simulink model "IEEE_39_bus_steady_state"  (R2021b)
settings: Solver=ode3  StartTime=0.0  StopTime=10  FixedStep=Ts  MaxStep=1/60  RelTol=1e-2  AbsTol=1e-1
PreLoadFcn:
  | Ts=50e-6; ssn_ieee39_params; dec=20;
InitFcn:
  | Ts=50e-6; ssn_ieee39_params; dec=20;
values from neighbouring files (symbols this model uses):
  f = 50    [ssn_ieee39_params_ctrl.m]
  fNom = f    (= 60)    [ssn_ieee39_params_ctrl.m]
  ILR = 5.02    [ssn_ieee39_params_ctrl.m]
  IQMIN = 0.1    [ssn_ieee39_params_ctrl.m]
  ISCLIM = 1    [ssn_ieee39_params_ctrl.m]
  ITFpu = 1.10    (= 1.1)    [ssn_ieee39_params_ctrl.m]
  K = 1    [ssn_ieee39_params_ctrl.m]
  K1 = 1    [ssn_ieee39_params_ctrl.m]
  K2 = 2    [ssn_ieee39_params_ctrl.m]
  KCL = 1.04    [ssn_ieee39_params_ctrl.m]
  KFB = 0    [ssn_ieee39_params_ctrl.m]
  KFF = 1    [ssn_ieee39_params_ctrl.m]
  KFIX = 1    [ssn_ieee39_params_ctrl.m]
  KG = 1    [ssn_ieee39_params_ctrl.m]
  KIA = 59.91    [ssn_ieee39_params_ctrl.m]
  KIOEX = 0.0303    [ssn_ieee39_params_ctrl.m]
  KIUEX = 0.0303    [ssn_ieee39_params_ctrl.m]
  KIUOEX = 1    [ssn_ieee39_params_ctrl.m]
  KIUUEX = 1    [ssn_ieee39_params_ctrl.m]
  KLR = 22.47    [ssn_ieee39_params_ctrl.m]
  KM = 1    [ssn_ieee39_params_ctrl.m]
  KOEL = 0.24    [ssn_ieee39_params_ctrl.m]
  Kp = 1    [ssn_ieee39_params_ctrl.m]
  KPA = 30    [ssn_ieee39_params_ctrl.m]
  KPOEL = 1    [ssn_ieee39_params_ctrl.m]
  KPOEX = 0    [ssn_ieee39_params_ctrl.m]
  KPUEX = 0    [ssn_ieee39_params_ctrl.m]
  KSCALE = 0.319    [ssn_ieee39_params_ctrl.m]
  KUF = 0    [ssn_ieee39_params_ctrl.m]
  KUI = 0.001    [ssn_ieee39_params_ctrl.m]
  KUL = 0.24    [ssn_ieee39_params_ctrl.m]
  s = 10    [ssn_ieee39_params_ctrl.m]
  TA = 0.01    [ssn_ieee39_params_ctrl.m]
  Tadj = 0    [ssn_ieee39_params_ctrl.m]
  taps = [1 1 1.07 1.07 1.009 1.025 1 1.025 1.025 1.025]*1    [ssn_ieee39_params_ctrl.m]
  TF = 0.02    [ssn_ieee39_params_ctrl.m]
  TG = 0.024    [ssn_ieee39_params_ctrl.m]
  TINV = 0    [ssn_ieee39_params_ctrl.m]
  TIT = 0.1    [ssn_ieee39_params_ctrl.m]
  TL_10_11_len = 14    [ssn_ieee39_params_ctrl.m]
  TL_10_13_len = 14    [ssn_ieee39_params_ctrl.m]
  TL_13_14_len = 32    [ssn_ieee39_params_ctrl.m]
  TL_14_15_len = 70    [ssn_ieee39_params_ctrl.m]
  TL_15_16_len = 31.5    [ssn_ieee39_params_ctrl.m]
  TL_16_17_len = 26    [ssn_ieee39_params_ctrl.m]
  TL_16_19_len = 61    [ssn_ieee39_params_ctrl.m]
  TL_16_21_len = 46    [ssn_ieee39_params_ctrl.m]
  TL_16_24_len = 15    [ssn_ieee39_params_ctrl.m]
  TL_17_18_len = 26    [ssn_ieee39_params_ctrl.m]
  TL_17_27_len = 59    [ssn_ieee39_params_ctrl.m]
  TL_1_2_len = 134    [ssn_ieee39_params_ctrl.m]
  TL_1_39_len = 105    [ssn_ieee39_params_ctrl.m]
  TL_21_22_len = 47    [ssn_ieee39_params_ctrl.m]
  TL_22_23_len = 33    [ssn_ieee39_params_ctrl.m]
  TL_24_23_len = 88    [ssn_ieee39_params_ctrl.m]
  TL_25_26_len = 101    [ssn_ieee39_params_ctrl.m]
  TL_26_27_len = 46.5    [ssn_ieee39_params_ctrl.m]
  TL_26_28_len = 151    [ssn_ieee39_params_ctrl.m]
  TL_26_29_len = 200    [ssn_ieee39_params_ctrl.m]
  TL_28_29_len = 48    [ssn_ieee39_params_ctrl.m]
  TL_2_25_len = 28    [ssn_ieee39_params_ctrl.m]
  TL_2_2_len = 49    [ssn_ieee39_params_ctrl.m]
  TL_3_18_len = 42    [ssn_ieee39_params_ctrl.m]
  TL_3_4_len = 53    [ssn_ieee39_params_ctrl.m]
  TL_4_14_len = 33    [ssn_ieee39_params_ctrl.m]
  TL_4_5_len = 32.5    [ssn_ieee39_params_ctrl.m]
  TL_5_6_len = 14    [ssn_ieee39_params_ctrl.m]
  TL_5_8_len = 32    [ssn_ieee39_params_ctrl.m]
  TL_6_11_len = 26.5    [ssn_ieee39_params_ctrl.m]
  TL_6_7_len = 25.5    [ssn_ieee39_params_ctrl.m]
  TL_7_8_len = 15    [ssn_ieee39_params_ctrl.m]
  TL_8_9_len = 93    [ssn_ieee39_params_ctrl.m]
  TL_9_39_len = 136    [ssn_ieee39_params_ctrl.m]
  TOEL = 5.00    (= 5)    [ssn_ieee39_params_ctrl.m]
  TQREF = 0    [ssn_ieee39_params_ctrl.m]
  TQSCL = 0.012    [ssn_ieee39_params_ctrl.m]
  Ts_PMU = 1/1000    (= 0.001)    [ssn_ieee39_params_ctrl.m]
  TU1 = 0    [ssn_ieee39_params_ctrl.m]
  TU2 = 0    [ssn_ieee39_params_ctrl.m]
  TU3 = 0    [ssn_ieee39_params_ctrl.m]
  TU4 = 0    [ssn_ieee39_params_ctrl.m]
  TUL = 0    [ssn_ieee39_params_ctrl.m]
  TUP = 0.050    (= 0.05)    [ssn_ieee39_params_ctrl.m]
  TUQ = .005    (= 0.005)    [ssn_ieee39_params_ctrl.m]
  TUV = 0.2    [ssn_ieee39_params_ctrl.m]
  VAAMAX = VAMAX    (= 7.05)    [ssn_ieee39_params_ctrl.m]
  VAMAX = 7.05    [ssn_ieee39_params_ctrl.m]
  VAMIN = -6.11    [ssn_ieee39_params_ctrl.m]
  VBMAX = 999    [ssn_ieee39_params_ctrl.m]
  VF = 0    [ssn_ieee39_params_ctrl.m]
  VFB = 0    [ssn_ieee39_params_ctrl.m]
  VMMAX = 7.05    [ssn_ieee39_params_ctrl.m]
  VMMIN = -6.11    [ssn_ieee39_params_ctrl.m]
  VOELmax1 = 0.2353    [ssn_ieee39_params_ctrl.m]
  VOELmax2 = 0.0    (= 0)    [ssn_ieee39_params_ctrl.m]
  VOELmin1 = -0.24    [ssn_ieee39_params_ctrl.m]
  VOELmin2 = -1.0    (= -1)    [ssn_ieee39_params_ctrl.m]
  VRMAX = 7.05    [ssn_ieee39_params_ctrl.m]
  VRMIN = -6.11    [ssn_ieee39_params_ctrl.m]
  VSCLmax = 0.20    (= 0.2)    [ssn_ieee39_params_ctrl.m]
  VSCLmin = -0.10    (= -0.1)    [ssn_ieee39_params_ctrl.m]
  VUELmax1 = 1    [ssn_ieee39_params_ctrl.m]
  VUELmax2 = 1    [ssn_ieee39_params_ctrl.m]
  VUELmin1 = -1    [ssn_ieee39_params_ctrl.m]
  VUELmin2 = -1    [ssn_ieee39_params_ctrl.m]
  VUImax = 1    [ssn_ieee39_params_ctrl.m]
  VUImin = -1    [ssn_ieee39_params_ctrl.m]
undefined symbols (not defined in the file or in its folder): D1, Delta, MOV_segment9, powergui
libraries: spsThreePhaseVIMeasurementLib x43, slpidlib x40, op_dpl_lib x32, powerlib_extras x30, simulink_extras x20, spsST2AModel x20, spsThreePhaseParallelRLCLoadLib x20, spsThreePhaseTransformerTwoWindingsLib x13, spsSynchronousMachinepuStandardLib x10, simulink x10, spsPower3phInstantaneousLib x10, spsThreePhasePISectionLineLib x4
(part 3 of 15)

== system IEEE_39_bus_steady_state/powergui ==
  note: Graphical user interface for the analysis of
      | Simscape Power Systems (Specialized Technology) circuits.
      | Place the Powergui block in the top-level of your model and double-click
      | on it to open the GUI.
  EquivalentModel1 : Subsystem
      mask init:
      | S  = GetDataForEquivalentModel('Discrete',gcbh);
      mask Display:
      | color('red')
      | disp('EQUIVALENT CIRCUIT\nDiscrete')
  EquivalentModel10 : Subsystem
      mask init:
      | S  = GetDataForEquivalentModel('Discrete',gcbh);
      mask Display:
      | color('red')
      | disp('EQUIVALENT CIRCUIT\nDiscrete')
  EquivalentModel11 : Subsystem
      mask init:
      | S  = GetDataForEquivalentModel('Discrete',gcbh);
      mask Display:
      | color('red')
      | disp('EQUIVALENT CIRCUIT\nDiscrete')
  EquivalentModel12 : Subsystem
      mask init:
      | S  = GetDataForEquivalentModel('Discrete',gcbh);
      mask Display:
      | color('red')
      | disp('EQUIVALENT CIRCUIT\nDiscrete')
  EquivalentModel13 : Subsystem
      mask init:
      | S  = GetDataForEquivalentModel('Discrete',gcbh);
      mask Display:
      | color('red')
      | disp('EQUIVALENT CIRCUIT\nDiscrete')
  EquivalentModel14 : Subsystem
      mask init:
      | S  = GetDataForEquivalentModel('Discrete',gcbh);
      mask Display:
      | color('red')
      | disp('EQUIVALENT CIRCUIT\nDiscrete')
  EquivalentModel15 : Subsystem
      mask init:
      | S  = GetDataForEquivalentModel('Discrete',gcbh);
      mask Display:
      | color('red')
      | disp('EQUIVALENT CIRCUIT\nDiscrete')
  EquivalentModel16 : Subsystem
      mask init:
      | S  = GetDataForEquivalentModel('Discrete',gcbh);
      mask Display:
      | color('red')
      | disp('EQUIVALENT CIRCUIT\nDiscrete')
  EquivalentModel17 : Subsystem
      mask init:
      | S  = GetDataForEquivalentModel('Discrete',gcbh);
      mask Display:
      | color('red')
      | disp('EQUIVALENT CIRCUIT\nDiscrete')
  EquivalentModel18 : Subsystem
      mask init:
      | S  = GetDataForEquivalentModel('Discrete',gcbh);
      mask Display:
      | color('red')
      | disp('EQUIVALENT CIRCUIT\nDiscrete')
  EquivalentModel19 : Subsystem
      mask init:
      | S  = GetDataForEquivalentModel('Discrete',gcbh);
      mask Display:
      | color('red')
      | disp('EQUIVALENT CIRCUIT\nDiscrete')
  EquivalentModel2 : Subsystem
      mask init:
      | S  = GetDataForEquivalentModel('Discrete',gcbh);
      mask Display:
      | color('red')
      | disp('EQUIVALENT CIRCUIT\nDiscrete')
  EquivalentModel20 : Subsystem
      mask init:
      | S  = GetDataForEquivalentModel('Discrete',gcbh);
      mask Display:
      | color('red')
      | disp('EQUIVALENT CIRCUIT\nDiscrete')
  EquivalentModel21 : Subsystem
      mask init:
      | S  = GetDataForEquivalentModel('Discrete',gcbh);
      mask Display:
      | color('red')
      | disp('EQUIVALENT CIRCUIT\nDiscrete')
  EquivalentModel22 : Subsystem
      mask init:
      | S  = GetDataForEquivalentModel('Discrete',gcbh);
      mask Display:
      | color('red')
      | disp('EQUIVALENT CIRCUIT\nDiscrete')
  EquivalentModel23 : Subsystem
      mask init:
      | S  = GetDataForEquivalentModel('Discrete',gcbh);
      mask Display:
      | color('red')
      | disp('EQUIVALENT CIRCUIT\nDiscrete')
  EquivalentModel24 : Subsystem
      mask init:
      | S  = GetDataForEquivalentModel('Discrete',gcbh);
      mask Display:
      | color('red')
      | disp('EQUIVALENT CIRCUIT\nDiscrete')
  EquivalentModel25 : Subsystem
      mask init:
      | S  = GetDataForEquivalentModel('Discrete',gcbh);
      mask Display:
      | color('red')
      | disp('EQUIVALENT CIRCUIT\nDiscrete')
  EquivalentModel26 : Subsystem
      mask init:
      | S  = GetDataForEquivalentModel('Discrete',gcbh);
      mask Display:
      | color('red')
      | disp('EQUIVALENT CIRCUIT\nDiscrete')
  EquivalentModel3 : Subsystem
      mask init:
      | S  = GetDataForEquivalentModel('Discrete',gcbh);
      mask Display:
      | color('red')
      | disp('EQUIVALENT CIRCUIT\nDiscrete')
  EquivalentModel4 : Subsystem
      mask init:
      | S  = GetDataForEquivalentModel('Discrete',gcbh);
      mask Display:
      | color('red')
      | disp('EQUIVALENT CIRCUIT\nDiscrete')
  EquivalentModel5 : Subsystem
      mask init:
      | S  = GetDataForEquivalentModel('Discrete',gcbh);
      mask Display:
      | color('red')
      | disp('EQUIVALENT CIRCUIT\nDiscrete')
  EquivalentModel6 : Subsystem
      mask init:
      | S  = GetDataForEquivalentModel('Discrete',gcbh);
      mask Display:
      | color('red')
      | disp('EQUIVALENT CIRCUIT\nDiscrete')
  EquivalentModel7 : Subsystem
      mask init:
      | S  = GetDataForEquivalentModel('Discrete',gcbh);
      mask Display:
      | color('red')
      | disp('EQUIVALENT CIRCUIT\nDiscrete')
  EquivalentModel8 : Subsystem
      mask init:
      | S  = GetDataForEquivalentModel('Discrete',gcbh);
      mask Display:
      | color('red')
      | disp('EQUIVALENT CIRCUIT\nDiscrete')
  EquivalentModel9 : Subsystem
      mask init:
      | S  = GetDataForEquivalentModel('Discrete',gcbh);
      mask Display:
      | color('red')
      | disp('EQUIVALENT CIRCUIT\nDiscrete')
  Ground : Ground
  Terminator : Terminator
  wires:
  Ground/1 -> Terminator/1

== system IEEE_39_bus_steady_state/SM_master/G1 ==
  Constant10 : Constant
  Constant6 : Constant
  G1 : Subsystem  AncestorBlock=|  mask(Diesel Generator (Simple)){Pn=1000e6, Vn=20e3, Fn=f, genType=PV, PQ0=[1 0.0], H1=6.54}
      | microgridLibrary/Diesel Generator
      | (GOV, AVR only)
      mask prompts: Pn "Generator Rated Power [W]"; Vn "Rated Voltage [V]"; Fn "Rated Frequency [Hz]"; genType "Load Flow Type"; PQ0 "Initial Power, [P0 Q0] [pu]"; H1 "Inertia Co-efficients [H(s)]"
      mask help:
      | The Diesel Generator block contains a synchronous generator, diesel governor and excitation system to represent the dynamics of a Genset. To inspect the model, look under the block mask (Ctrl + u).
      |
      | The inputs to the basic Diesel generator block are the desired speed reference (in pu) and the desired voltage reference (in pu). The output measurements are contained in a Simulink bus, which can be selected by using the Bus Selector block.
      |
      | Note: The initial generator power must be specified for use for Load Flow analysis.
      mask init:
      | % Extract Initial Active/Reactive Power
      | P0 = PQ0(1);
      | Q0 = PQ0(2);
      | 
      | % Select Load Flow Type
      | genBlock = [gcb '/Synchronous Machine'];
      | currentVals = get_param(genBlock,'MaskValues');
      | currentVals{31} = genType;
      | set_param(genBlock,'MaskValues',currentVals);
      | 
      | % Disable Option if Swing Generator Selected
      | currentEnables = get_param(gcb,'MaskEnables');
      | if strcmp(genType,'swing')
      |     currentEnables{5} = 'off';
      | else
      |     currentEnables{5} = 'on';
      | end
      | set_param(gcb,'MaskEnables',currentEnables);
      mask TypeOptions genType: swing | PQ | PV
      mask Display:
      | %image(imread('diesel.jpg'))
      | color('black')
      | port_label('input',1,'wref (pu)')
      | port_label('input',2,'Vref (pu)')
      | port_label('output',1,'m')
      | port_label('Rconn',1,'A')
      | port_label('Rconn',2,'B')
      | port_label('Rconn',3,'C')
  Terminator : Terminator
  C : PMIOPort  Side=Right
  B : PMIOPort  Port=2  Side=Right
  A : PMIOPort  Port=3  Side=Right
  wires:
  Constant10/1 -> G1/1(wref (pu))
  Constant6/1 -> G1/2(Vref (pu))
  G1/1(sm1) -> Terminator/1
  connections:
  G1/RConn1 -- A/RConn1
  G1/RConn3 -- C/RConn1
  G1/RConn2 -- B/RConn1

== system IEEE_39_bus_steady_state/SM_master/G10 ==
  Constant10 : Constant
  Constant6 : Constant
  G10 : Subsystem  AncestorBlock=|  mask(Diesel Generator (Simple)){Pn=1000e6, Vn=20e3, Fn=f, genType=PV, PQ0=[0.25 0.0], H1=6.54}
      | microgridLibrary/Diesel Generator
      | (GOV, AVR only)
      mask prompts: Pn "Generator Rated Power [W]"; Vn "Rated Voltage [V]"; Fn "Rated Frequency [Hz]"; genType "Load Flow Type"; PQ0 "Initial Power, [P0 Q0] [pu]"; H1 "Inertia Co-efficients [H(s)]"
      mask help:
      | The Diesel Generator block contains a synchronous generator, diesel governor and excitation system to represent the dynamics of a Genset. To inspect the model, look under the block mask (Ctrl + u).
      |
      | The inputs to the basic Diesel generator block are the desired speed reference (in pu) and the desired voltage reference (in pu). The output measurements are contained in a Simulink bus, which can be selected by using the Bus Selector block.
      |
      | Note: The initial generator power must be specified for use for Load Flow analysis.
      mask init: same as IEEE_39_bus_steady_state/SM_master/G1/G1
      mask TypeOptions genType: swing | PQ | PV
      mask Display:
      | %image(imread('diesel.jpg'))
      | color('black')
      | port_label('input',1,'wref (pu)')
      | port_label('input',2,'Vref (pu)')
      | port_label('output',1,'m')
      | port_label('Rconn',1,'A')
      | port_label('Rconn',2,'B')
      | port_label('Rconn',3,'C')
  Terminator : Terminator
  A : PMIOPort  Side=Right
  B : PMIOPort  Port=2  Side=Right
  C : PMIOPort  Port=3  Side=Right
  wires:
  G10/1(sm1) -> Terminator/1
  Constant6/1 -> G10/2(Vref (pu))
  Constant10/1 -> G10/1(wref (pu))
  connections:
  G10/RConn2 -- B/RConn1
  G10/RConn3 -- C/RConn1
  G10/RConn1 -- A/RConn1

== system IEEE_39_bus_steady_state/SM_master/G2 ==
  Constant10 : Constant
  Constant6 : Constant
  G2 : Subsystem  AncestorBlock=|  mask(Diesel Generator (Simple)){Pn=1000e6, Vn=20e3, Fn=f, genType=PV, PQ0=[0.2777 0.0], H1=6.54}
      | microgridLibrary/Diesel Generator
      | (GOV, AVR only)
      mask prompts: Pn "Generator Rated Power [W]"; Vn "Rated Voltage [V]"; Fn "Rated Frequency [Hz]"; genType "Load Flow Type"; PQ0 "Initial Power, [P0 Q0] [pu]"; H1 "Inertia Co-efficients [H(s)]"
      mask help:
      | The Diesel Generator block contains a synchronous generator, diesel governor and excitation system to represent the dynamics of a Genset. To inspect the model, look under the block mask (Ctrl + u).
      |
      | The inputs to the basic Diesel generator block are the desired speed reference (in pu) and the desired voltage reference (in pu). The output measurements are contained in a Simulink bus, which can be selected by using the Bus Selector block.
      |
      | Note: The initial generator power must be specified for use for Load Flow analysis.
      mask init: same as IEEE_39_bus_steady_state/SM_master/G1/G1
      mask TypeOptions genType: swing | PQ | PV
      mask Display:
      | %image(imread('diesel.jpg'))
      | color('black')
      | port_label('input',1,'wref (pu)')
      | port_label('input',2,'Vref (pu)')
      | port_label('output',1,'m')
      | port_label('Rconn',1,'A')
      | port_label('Rconn',2,'B')
      | port_label('Rconn',3,'C')
  Terminator : Terminator
  A : PMIOPort  Side=Right
  B : PMIOPort  Port=2  Side=Right
  C : PMIOPort  Port=3  Side=Right
  wires:
  Constant10/1 -> G2/1(wref (pu))
  Constant6/1 -> G2/2(Vref (pu))
  G2/1(sm1) -> Terminator/1
  connections:
  G2/RConn1 -- A/RConn1
  G2/RConn3 -- C/RConn1
  G2/RConn2 -- B/RConn1

== system IEEE_39_bus_steady_state/SM_master/G3 ==
  Constant10 : Constant
  Constant6 : Constant
  G3 : Subsystem  AncestorBlock=|  mask(Diesel Generator (Simple)){Pn=1000e6, Vn=20e3, Fn=f, genType=PV, PQ0=[0.65 0.0], H1=6.54}
      | microgridLibrary/Diesel Generator
      | (GOV, AVR only)
      mask prompts: Pn "Generator Rated Power [W]"; Vn "Rated Voltage [V]"; Fn "Rated Frequency [Hz]"; genType "Load Flow Type"; PQ0 "Initial Power, [P0 Q0] [pu]"; H1 "Inertia Co-efficients [H(s)]"
      mask help:
      | The Diesel Generator block contains a synchronous generator, diesel governor and excitation system to represent the dynamics of a Genset. To inspect the model, look under the block mask (Ctrl + u).
      |
      | The inputs to the basic Diesel generator block are the desired speed reference (in pu) and the desired voltage reference (in pu). The output measurements are contained in a Simulink bus, which can be selected by using the Bus Selector block.
      |
      | Note: The initial generator power must be specified for use for Load Flow analysis.
      mask init: same as IEEE_39_bus_steady_state/SM_master/G1/G1
      mask TypeOptions genType: swing | PQ | PV
      mask Display:
      | %image(imread('diesel.jpg'))
      | color('black')
      | port_label('input',1,'wref (pu)')
      | port_label('input',2,'Vref (pu)')
      | port_label('output',1,'m')
      | port_label('Rconn',1,'A')
      | port_label('Rconn',2,'B')
      | port_label('Rconn',3,'C')
  Terminator : Terminator
  A : PMIOPort  Side=Right
  B : PMIOPort  Port=2  Side=Right
  C : PMIOPort  Port=3  Side=Right
  wires:
  G3/1(sm1) -> Terminator/1
  Constant6/1 -> G3/2(Vref (pu))
  Constant10/1 -> G3/1(wref (pu))
  connections:
  G3/RConn2 -- B/RConn1
  G3/RConn3 -- C/RConn1
  G3/RConn1 -- A/RConn1

== system IEEE_39_bus_steady_state/SM_master/G4 ==
  Constant10 : Constant
  Constant6 : Constant
  G4 : Subsystem  AncestorBlock=|  mask(Diesel Generator (Simple)){Pn=1000e6, Vn=20e3, Fn=f, genType=PV, PQ0=[0.632 0.0], H1=6.54}
      | microgridLibrary/Diesel Generator
      | (GOV, AVR only)
      mask prompts: Pn "Generator Rated Power [W]"; Vn "Rated Voltage [V]"; Fn "Rated Frequency [Hz]"; genType "Load Flow Type"; PQ0 "Initial Power, [P0 Q0] [pu]"; H1 "Inertia Co-efficients [H(s)]"
      mask help:
      | The Diesel Generator block contains a synchronous generator, diesel governor and excitation system to represent the dynamics of a Genset. To inspect the model, look under the block mask (Ctrl + u).
      |
      | The inputs to the basic Diesel generator block are the desired speed reference (in pu) and the desired voltage reference (in pu). The output measurements are contained in a Simulink bus, which can be selected by using the Bus Selector block.
      |
      | Note: The initial generator power must be specified for use for Load Flow analysis.
      mask init: same as IEEE_39_bus_steady_state/SM_master/G1/G1
      mask TypeOptions genType: swing | PQ | PV
      mask Display:
      | %image(imread('diesel.jpg'))
      | color('black')
      | port_label('input',1,'wref (pu)')
      | port_label('input',2,'Vref (pu)')
      | port_label('output',1,'m')
      | port_label('Rconn',1,'A')
      | port_label('Rconn',2,'B')
      | port_label('Rconn',3,'C')
  Terminator : Terminator
  A : PMIOPort  Side=Right
  B : PMIOPort  Port=2  Side=Right
  C : PMIOPort  Port=3  Side=Right
  wires:
  G4/1(sm1) -> Terminator/1
  Constant6/1 -> G4/2(Vref (pu))
  Constant10/1 -> G4/1(wref (pu))
  connections:
  G4/RConn2 -- B/RConn1
  G4/RConn3 -- C/RConn1
  G4/RConn1 -- A/RConn1

== system IEEE_39_bus_steady_state/SM_master/G5 ==
  Constant10 : Constant
  Constant6 : Constant
  G5 : Subsystem  AncestorBlock=|  mask(Diesel Generator (Simple)){Pn=1000e6, Vn=20e3, Fn=f, genType=PV, PQ0=[0.504 0.0], H1=6.54}
      | microgridLibrary/Diesel Generator
      | (GOV, AVR only)
      mask prompts: Pn "Generator Rated Power [W]"; Vn "Rated Voltage [V]"; Fn "Rated Frequency [Hz]"; genType "Load Flow Type"; PQ0 "Initial Power, [P0 Q0] [pu]"; H1 "Inertia Co-efficients [H(s)]"
      mask help:
      | The Diesel Generator block contains a synchronous generator, diesel governor and excitation system to represent the dynamics of a Genset. To inspect the model, look under the block mask (Ctrl + u).
      |
      | The inputs to the basic Diesel generator block are the desired speed reference (in pu) and the desired voltage reference (in pu). The output measurements are contained in a Simulink bus, which can be selected by using the Bus Selector block.
      |
      | Note: The initial generator power must be specified for use for Load Flow analysis.
      mask init: same as IEEE_39_bus_steady_state/SM_master/G1/G1
      mask TypeOptions genType: swing | PQ | PV
      mask Display:
      | %image(imread('diesel.jpg'))
      | color('black')
      | port_label('input',1,'wref (pu)')
      | port_label('input',2,'Vref (pu)')
      | port_label('output',1,'m')
      | port_label('Rconn',1,'A')
      | port_label('Rconn',2,'B')
      | port_label('Rconn',3,'C')
  Terminator : Terminator
  A : PMIOPort  Side=Right
  B : PMIOPort  Port=2  Side=Right
  C : PMIOPort  Port=3  Side=Right
  wires:
  Constant10/1 -> G5/1(wref (pu))
  Constant6/1 -> G5/2(Vref (pu))
  G5/1(sm1) -> Terminator/1
  connections:
  G5/RConn1 -- A/RConn1
  G5/RConn3 -- C/RConn1
  G5/RConn2 -- B/RConn1

== system IEEE_39_bus_steady_state/SM_master/G6 ==
  Constant10 : Constant
  Constant6 : Constant
  G6 : Subsystem  AncestorBlock=|  mask(Diesel Generator (Simple)){Pn=1000e6, Vn=20e3, Fn=f, genType=PV, PQ0=[0.65 0.0], H1=6.54}
      | microgridLibrary/Diesel Generator
      | (GOV, AVR only)
      mask prompts: Pn "Generator Rated Power [W]"; Vn "Rated Voltage [V]"; Fn "Rated Frequency [Hz]"; genType "Load Flow Type"; PQ0 "Initial Power, [P0 Q0] [pu]"; H1 "Inertia Co-efficients [H(s)]"
      mask help:
      | The Diesel Generator block contains a synchronous generator, diesel governor and excitation system to represent the dynamics of a Genset. To inspect the model, look under the block mask (Ctrl + u).
      |
      | The inputs to the basic Diesel generator block are the desired speed reference (in pu) and the desired voltage reference (in pu). The output measurements are contained in a Simulink bus, which can be selected by using the Bus Selector block.
      |
      | Note: The initial generator power must be specified for use for Load Flow analysis.
      mask init: same as IEEE_39_bus_steady_state/SM_master/G1/G1
      mask TypeOptions genType: swing | PQ | PV
      mask Display:
      | %image(imread('diesel.jpg'))
      | color('black')
      | port_label('input',1,'wref (pu)')
      | port_label('input',2,'Vref (pu)')
      | port_label('output',1,'m')
      | port_label('Rconn',1,'A')
      | port_label('Rconn',2,'B')
      | port_label('Rconn',3,'C')
  Terminator : Terminator
  A : PMIOPort  Side=Right
  B : PMIOPort  Port=2  Side=Right
  C : PMIOPort  Port=3  Side=Right
  wires:
  G6/1(sm1) -> Terminator/1
  Constant6/1 -> G6/2(Vref (pu))
  Constant10/1 -> G6/1(wref (pu))
  connections:
  G6/RConn2 -- B/RConn1
  G6/RConn3 -- C/RConn1
  G6/RConn1 -- A/RConn1

== system IEEE_39_bus_steady_state/SM_master/G7 ==
  Constant10 : Constant
  Constant6 : Constant
  G7 : Subsystem  AncestorBlock=|  mask(Diesel Generator (Simple)){Pn=1000e6, Vn=20e3, Fn=f, genType=PV, PQ0=[0.56 0.0], H1=6.54}
      | microgridLibrary/Diesel Generator
      | (GOV, AVR only)
      mask prompts: Pn "Generator Rated Power [W]"; Vn "Rated Voltage [V]"; Fn "Rated Frequency [Hz]"; genType "Load Flow Type"; PQ0 "Initial Power, [P0 Q0] [pu]"; H1 "Inertia Co-efficients [H(s)]"
      mask help:
      | The Diesel Generator block contains a synchronous generator, diesel governor and excitation system to represent the dynamics of a Genset. To inspect the model, look under the block mask (Ctrl + u).
      |
      | The inputs to the basic Diesel generator block are the desired speed reference (in pu) and the desired voltage reference (in pu). The output measurements are contained in a Simulink bus, which can be selected by using the Bus Selector block.
      |
      | Note: The initial generator power must be specified for use for Load Flow analysis.
      mask init: same as IEEE_39_bus_steady_state/SM_master/G1/G1
      mask TypeOptions genType: swing | PQ | PV
      mask Display:
      | %image(imread('diesel.jpg'))
      | color('black')
      | port_label('input',1,'wref (pu)')
      | port_label('input',2,'Vref (pu)')
      | port_label('output',1,'m')
      | port_label('Rconn',1,'A')
      | port_label('Rconn',2,'B')
      | port_label('Rconn',3,'C')
  Terminator : Terminator
  A : PMIOPort  Side=Right
  B : PMIOPort  Port=2  Side=Right
  C : PMIOPort  Port=3  Side=Right
  wires:
  G7/1(sm1) -> Terminator/1
  Constant6/1 -> G7/2(Vref (pu))
  Constant10/1 -> G7/1(wref (pu))
  connections:
  G7/RConn2 -- B/RConn1
  G7/RConn3 -- C/RConn1
  G7/RConn1 -- A/RConn1

== system IEEE_39_bus_steady_state/SM_master/G8 ==
  " G8" : Subsystem  AncestorBlock=|  mask(Diesel Generator (Simple)){Pn=1000e6, Vn=20e3, Fn=f, genType=PV, PQ0=[0.54 0.0], H1=6.54}
      | microgridLibrary/Diesel Generator
      | (GOV, AVR only)
      mask prompts: Pn "Generator Rated Power [W]"; Vn "Rated Voltage [V]"; Fn "Rated Frequency [Hz]"; genType "Load Flow Type"; PQ0 "Initial Power, [P0 Q0] [pu]"; H1 "Inertia Co-efficients [H(s)]"
      mask help:
      | The Diesel Generator block contains a synchronous generator, diesel governor and excitation system to represent the dynamics of a Genset. To inspect the model, look under the block mask (Ctrl + u).
      |
      | The inputs to the basic Diesel generator block are the desired speed reference (in pu) and the desired voltage reference (in pu). The output measurements are contained in a Simulink bus, which can be selected by using the Bus Selector block.
      |
      | Note: The initial generator power must be specified for use for Load Flow analysis.
      mask init: same as IEEE_39_bus_steady_state/SM_master/G1/G1
      mask TypeOptions genType: swing | PQ | PV
      mask Display:
      | %image(imread('diesel.jpg'))
      | color('black')
      | port_label('input',1,'wref (pu)')
      | port_label('input',2,'Vref (pu)')
      | port_label('output',1,'m')
      | port_label('Rconn',1,'A')
      | port_label('Rconn',2,'B')
      | port_label('Rconn',3,'C')
  Constant10 : Constant
  Constant6 : Constant
  Terminator : Terminator
  A : PMIOPort  Side=Right
  B : PMIOPort  Port=2  Side=Right
  C : PMIOPort  Port=3  Side=Right
  wires:
  Constant10/1 -> " G8"/1(wref (pu))
  Constant6/1 -> " G8"/2(Vref (pu))
  " G8"/1(sm1) -> Terminator/1
  connections:
  " G8"/RConn1 -- A/RConn1
  " G8"/RConn3 -- C/RConn1
  " G8"/RConn2 -- B/RConn1

== system IEEE_39_bus_steady_state/SM_master/G9 ==
  Constant10 : Constant
  Constant6 : Constant
  G9 : Subsystem  AncestorBlock=|  mask(Diesel Generator (Simple)){Pn=1000e6, Vn=20e3, Fn=f, genType=PV, PQ0=[0.83 0.0], H1=6.54}
      | microgridLibrary/Diesel Generator
      | (GOV, AVR only)
      mask prompts: Pn "Generator Rated Power [W]"; Vn "Rated Voltage [V]"; Fn "Rated Frequency [Hz]"; genType "Load Flow Type"; PQ0 "Initial Power, [P0 Q0] [pu]"; H1 "Inertia Co-efficients [H(s)]"
      mask help:
      | The Diesel Generator block contains a synchronous generator, diesel governor and excitation system to represent the dynamics of a Genset. To inspect the model, look under the block mask (Ctrl + u).
      |
      | The inputs to the basic Diesel generator block are the desired speed reference (in pu) and the desired voltage reference (in pu). The output measurements are contained in a Simulink bus, which can be selected by using the Bus Selector block.
      |
      | Note: The initial generator power must be specified for use for Load Flow analysis.
      mask init: same as IEEE_39_bus_steady_state/SM_master/G1/G1
      mask TypeOptions genType: swing | PQ | PV
      mask Display:
      | %image(imread('diesel.jpg'))
      | color('black')
      | port_label('input',1,'wref (pu)')
      | port_label('input',2,'Vref (pu)')
      | port_label('output',1,'m')
      | port_label('Rconn',1,'A')
      | port_label('Rconn',2,'B')
      | port_label('Rconn',3,'C')
  Terminator : Terminator
  A : PMIOPort  Side=Right
  B : PMIOPort  Port=2  Side=Right
  C : PMIOPort  Port=3  Side=Right
  wires:
  G9/1(sm1) -> Terminator/1
  Constant6/1 -> G9/2(Vref (pu))
  Constant10/1 -> G9/1(wref (pu))
  connections:
  G9/RConn2 -- B/RConn1
  G9/RConn3 -- C/RConn1
  G9/RConn1 -- A/RConn1

== system IEEE_39_bus_steady_state/SM_master/PMU_Vpos_60Hz ==
  abc : Inport  PortDimensions=3
  1 / sqrt of 2 : Gain  Gain=1/sqrt(2)  OutDataTypeStr=Inherit: Same as input  ParamDataTypeStr=Inherit: Same as input
  Cartesian to Polar : simulink_extras/Transformations/Cartesian to Polar
  Demux : Demux  Outputs=3
      settings: DisplayOption=none
  Discrete Mean value1 : powerlib_extras/Discrete Measurements/Discrete  Mean value  Freq=Freq  Vinit=Real_Init  Ts=Ts
      settings: SourceProductBaseCode=PS
  Discrete Mean value2 : powerlib_extras/Discrete Measurements/Discrete  Mean value  Freq=Freq  Vinit=Imag_Init  Ts=Ts
      settings: SourceProductBaseCode=PS
  Discrete Derivative : simulink/Discrete/Discrete Derivative  gainval=1.0  ICPrevScaledInput=0.0  OutMin=[]  OutMax=[]  OutDataType=fixdt(1, 16)  OutScaling=2^-10  DoSatur=off
  Gain : Gain  Gain=2*pi*Freq  SaturateOnIntegerOverflow=on  OutDataTypeStr=Inherit: Same as input  ParamDataTypeStr=Inherit: Same as input
  Mux : Mux  Inputs=2
  Rad->Deg. : Gain  Gain=180/pi  SaturateOnIntegerOverflow=on  OutDataTypeStr=Inherit: Same as input  ParamDataTypeStr=Inherit: Same as input
  Sum : Sum  Inputs=|++  OutDataTypeStr=Inherit: Same as first input
  Terminator : Terminator
  Trigonometric Function : Trigonometry
  Trigonometric Function1 : Trigonometry  Operator=cos
  abc_to_dq0 Transformation : powerlib_extras/Measurements/abc_to_dq0 Transformation
      settings: SourceProductBaseCode=PS
  fo : Constant  Value=2*pi*Freq
  t : DigitalClock  SampleTime=Ts
  Mag : Outport
  Phase : Outport  Port=2
  freq : Outport  Port=3
  dfdt : Outport  Port=4
  wires:
  Cartesian to Polar/2 -> Rad->Deg./1, Discrete Derivative/1
  Gain/1 -> Trigonometric Function1/1, Trigonometric Function/1
  t/1 -> Gain/1
  abc/1 -> abc_to_dq0 Transformation/1
  Mux/1 -> abc_to_dq0 Transformation/2
  Discrete Mean value1/1 -> Cartesian to Polar/1  "Real"
  Rad->Deg./1 -> Phase/1
  Discrete Mean value2/1 -> Cartesian to Polar/2  "Real"
  abc_to_dq0 Transformation/1 -> Demux/1
  Demux/3 -> Terminator/1
  Demux/2 -> Discrete Mean value2/1
  Demux/1 -> Discrete Mean value1/1
  Trigonometric Function/1 -> Mux/1
  Trigonometric Function1/1 -> Mux/2
  Cartesian to Polar/1 -> 1 / sqrt of 2/1
  1 / sqrt of 2/1 -> Mag/1
  Discrete Derivative/1 -> Sum/2, dfdt/1
  fo/1 -> Sum/1
  Sum/1 -> freq/1

== system IEEE_39_bus_steady_state/SM_master/PMU_Vpos_60Hz1 ==
  abc : Inport  PortDimensions=3
  1 / sqrt of 2 : Gain  Gain=1/sqrt(2)  OutDataTypeStr=Inherit: Same as input  ParamDataTypeStr=Inherit: Same as input
  Cartesian to Polar : simulink_extras/Transformations/Cartesian to Polar
  Demux : Demux  Outputs=3
      settings: DisplayOption=none
  Discrete Mean value1 : powerlib_extras/Discrete Measurements/Discrete  Mean value  Freq=Freq  Vinit=Real_Init  Ts=Ts
      settings: SourceProductBaseCode=PS
  Discrete Mean value2 : powerlib_extras/Discrete Measurements/Discrete  Mean value  Freq=Freq  Vinit=Imag_Init  Ts=Ts
      settings: SourceProductBaseCode=PS
  Discrete Derivative : simulink/Discrete/Discrete Derivative  gainval=1.0  ICPrevScaledInput=0.0  OutMin=[]  OutMax=[]  OutDataType=fixdt(1, 16)  OutScaling=2^-10  DoSatur=off
  Gain : Gain  Gain=2*pi*Freq  SaturateOnIntegerOverflow=on  OutDataTypeStr=Inherit: Same as input  ParamDataTypeStr=Inherit: Same as input
  Mux : Mux  Inputs=2
  Rad->Deg. : Gain  Gain=180/pi  SaturateOnIntegerOverflow=on  OutDataTypeStr=Inherit: Same as input  ParamDataTypeStr=Inherit: Same as input
  Sum : Sum  Inputs=|++  OutDataTypeStr=Inherit: Same as first input
  Terminator : Terminator
  Trigonometric Function : Trigonometry
  Trigonometric Function1 : Trigonometry  Operator=cos
  abc_to_dq0 Transformation : powerlib_extras/Measurements/abc_to_dq0 Transformation
      settings: SourceProductBaseCode=PS
  fo : Constant  Value=2*pi*Freq
  t : DigitalClock  SampleTime=Ts
  Mag : Outport
  Phase : Outport  Port=2
  freq : Outport  Port=3
  dfdt : Outport  Port=4
  wires:
  Cartesian to Polar/2 -> Rad->Deg./1, Discrete Derivative/1
  Gain/1 -> Trigonometric Function1/1, Trigonometric Function/1
  t/1 -> Gain/1
  abc/1 -> abc_to_dq0 Transformation/1
  Mux/1 -> abc_to_dq0 Transformation/2
  Discrete Mean value1/1 -> Cartesian to Polar/1  "Real"
  Rad->Deg./1 -> Phase/1
  Discrete Mean value2/1 -> Cartesian to Polar/2  "Real"
  abc_to_dq0 Transformation/1 -> Demux/1
  Demux/3 -> Terminator/1
  Demux/2 -> Discrete Mean value2/1
  Demux/1 -> Discrete Mean value1/1
  Trigonometric Function/1 -> Mux/1
  Trigonometric Function1/1 -> Mux/2
  Cartesian to Polar/1 -> 1 / sqrt of 2/1
  1 / sqrt of 2/1 -> Mag/1
  Discrete Derivative/1 -> Sum/2, dfdt/1
  fo/1 -> Sum/1
  Sum/1 -> freq/1

== system IEEE_39_bus_steady_state/SM_master/PMU_Vpos_60Hz2 ==
  abc : Inport  PortDimensions=3
  1 / sqrt of 2 : Gain  Gain=1/sqrt(2)  OutDataTypeStr=Inherit: Same as input  ParamDataTypeStr=Inherit: Same as input
  Cartesian to Polar : simulink_extras/Transformations/Cartesian to Polar
  Demux : Demux  Outputs=3
      settings: DisplayOption=none
  Discrete Mean value1 : powerlib_extras/Discrete Measurements/Discrete  Mean value  Freq=Freq  Vinit=Real_Init  Ts=Ts
      settings: SourceProductBaseCode=PS
  Discrete Mean value2 : powerlib_extras/Discrete Measurements/Discrete  Mean value  Freq=Freq  Vinit=Imag_Init  Ts=Ts
      settings: SourceProductBaseCode=PS
  Discrete Derivative : simulink/Discrete/Discrete Derivative  gainval=1.0  ICPrevScaledInput=0.0  OutMin=[]  OutMax=[]  OutDataType=fixdt(1, 16)  OutScaling=2^-10  DoSatur=off
  Gain : Gain  Gain=2*pi*Freq  SaturateOnIntegerOverflow=on  OutDataTypeStr=Inherit: Same as input  ParamDataTypeStr=Inherit: Same as input
  Mux : Mux  Inputs=2
  Rad->Deg. : Gain  Gain=180/pi  SaturateOnIntegerOverflow=on  OutDataTypeStr=Inherit: Same as input  ParamDataTypeStr=Inherit: Same as input
  Sum : Sum  Inputs=|++  OutDataTypeStr=Inherit: Same as first input
  Terminator : Terminator
  Trigonometric Function : Trigonometry
  Trigonometric Function1 : Trigonometry  Operator=cos
  abc_to_dq0 Transformation : powerlib_extras/Measurements/abc_to_dq0 Transformation
      settings: SourceProductBaseCode=PS
  fo : Constant  Value=2*pi*Freq
  t : DigitalClock  SampleTime=Ts
  Mag : Outport
  Phase : Outport  Port=2
  freq : Outport  Port=3
  dfdt : Outport  Port=4
  wires:
  Cartesian to Polar/2 -> Rad->Deg./1, Discrete Derivative/1
  Gain/1 -> Trigonometric Function1/1, Trigonometric Function/1
  t/1 -> Gain/1
  abc/1 -> abc_to_dq0 Transformation/1
  Mux/1 -> abc_to_dq0 Transformation/2
  Discrete Mean value1/1 -> Cartesian to Polar/1  "Real"
  Rad->Deg./1 -> Phase/1
  Discrete Mean value2/1 -> Cartesian to Polar/2  "Real"
  abc_to_dq0 Transformation/1 -> Demux/1
  Demux/3 -> Terminator/1
  Demux/2 -> Discrete Mean value2/1
  Demux/1 -> Discrete Mean value1/1
  Trigonometric Function/1 -> Mux/1
  Trigonometric Function1/1 -> Mux/2
  Cartesian to Polar/1 -> 1 / sqrt of 2/1
  1 / sqrt of 2/1 -> Mag/1
  Discrete Derivative/1 -> Sum/2, dfdt/1
  fo/1 -> Sum/1
  Sum/1 -> freq/1

== system IEEE_39_bus_steady_state/SM_master/PMU_Vpos_60Hz3 ==
  abc : Inport  PortDimensions=3
  1 / sqrt of 2 : Gain  Gain=1/sqrt(2)  OutDataTypeStr=Inherit: Same as input  ParamDataTypeStr=Inherit: Same as input
  Cartesian to Polar : simulink_extras/Transformations/Cartesian to Polar
  Demux : Demux  Outputs=3
      settings: DisplayOption=none
  Discrete Mean value1 : powerlib_extras/Discrete Measurements/Discrete  Mean value  Freq=Freq  Vinit=Real_Init  Ts=Ts
      settings: SourceProductBaseCode=PS
  Discrete Mean value2 : powerlib_extras/Discrete Measurements/Discrete  Mean value  Freq=Freq  Vinit=Imag_Init  Ts=Ts
      settings: SourceProductBaseCode=PS
  Discrete Derivative : simulink/Discrete/Discrete Derivative  gainval=1.0  ICPrevScaledInput=0.0  OutMin=[]  OutMax=[]  OutDataType=fixdt(1, 16)  OutScaling=2^-10  DoSatur=off
  Gain : Gain  Gain=2*pi*Freq  SaturateOnIntegerOverflow=on  OutDataTypeStr=Inherit: Same as input  ParamDataTypeStr=Inherit: Same as input
  Mux : Mux  Inputs=2
  Rad->Deg. : Gain  Gain=180/pi  SaturateOnIntegerOverflow=on  OutDataTypeStr=Inherit: Same as input  ParamDataTypeStr=Inherit: Same as input
  Sum : Sum  Inputs=|++  OutDataTypeStr=Inherit: Same as first input
  Terminator : Terminator
  Trigonometric Function : Trigonometry
  Trigonometric Function1 : Trigonometry  Operator=cos
  abc_to_dq0 Transformation : powerlib_extras/Measurements/abc_to_dq0 Transformation
      settings: SourceProductBaseCode=PS
  fo : Constant  Value=2*pi*Freq
  t : DigitalClock  SampleTime=Ts
  Mag : Outport
  Phase : Outport  Port=2
  freq : Outport  Port=3
  dfdt : Outport  Port=4
  wires:
  Cartesian to Polar/2 -> Rad->Deg./1, Discrete Derivative/1
  Gain/1 -> Trigonometric Function1/1, Trigonometric Function/1
  t/1 -> Gain/1
  abc/1 -> abc_to_dq0 Transformation/1
  Mux/1 -> abc_to_dq0 Transformation/2
  Discrete Mean value1/1 -> Cartesian to Polar/1  "Real"
  Rad->Deg./1 -> Phase/1
  Discrete Mean value2/1 -> Cartesian to Polar/2  "Real"
  abc_to_dq0 Transformation/1 -> Demux/1
  Demux/3 -> Terminator/1
  Demux/2 -> Discrete Mean value2/1
  Demux/1 -> Discrete Mean value1/1
  Trigonometric Function/1 -> Mux/1
  Trigonometric Function1/1 -> Mux/2
  Cartesian to Polar/1 -> 1 / sqrt of 2/1
  1 / sqrt of 2/1 -> Mag/1
  Discrete Derivative/1 -> Sum/2, dfdt/1
  fo/1 -> Sum/1
  Sum/1 -> freq/1

== system IEEE_39_bus_steady_state/SM_master/PMU_Vpos_60Hz4 ==
  abc : Inport  PortDimensions=3
  1 / sqrt of 2 : Gain  Gain=1/sqrt(2)  OutDataTypeStr=Inherit: Same as input  ParamDataTypeStr=Inherit: Same as input
  Cartesian to Polar : simulink_extras/Transformations/Cartesian to Polar
  Demux : Demux  Outputs=3
      settings: DisplayOption=none
  Discrete Mean value1 : powerlib_extras/Discrete Measurements/Discrete  Mean value  Freq=Freq  Vinit=Real_Init  Ts=Ts
      settings: SourceProductBaseCode=PS
  Discrete Mean value2 : powerlib_extras/Discrete Measurements/Discrete  Mean value  Freq=Freq  Vinit=Imag_Init  Ts=Ts
      settings: SourceProductBaseCode=PS
  Discrete Derivative : simulink/Discrete/Discrete Derivative  gainval=1.0  ICPrevScaledInput=0.0  OutMin=[]  OutMax=[]  OutDataType=fixdt(1, 16)  OutScaling=2^-10  DoSatur=off
  Gain : Gain  Gain=2*pi*Freq  SaturateOnIntegerOverflow=on  OutDataTypeStr=Inherit: Same as input  ParamDataTypeStr=Inherit: Same as input
  Mux : Mux  Inputs=2
  Rad->Deg. : Gain  Gain=180/pi  SaturateOnIntegerOverflow=on  OutDataTypeStr=Inherit: Same as input  ParamDataTypeStr=Inherit: Same as input
  Sum : Sum  Inputs=|++  OutDataTypeStr=Inherit: Same as first input
  Terminator : Terminator
  Trigonometric Function : Trigonometry
  Trigonometric Function1 : Trigonometry  Operator=cos
  abc_to_dq0 Transformation : powerlib_extras/Measurements/abc_to_dq0 Transformation
      settings: SourceProductBaseCode=PS
  fo : Constant  Value=2*pi*Freq
  t : DigitalClock  SampleTime=Ts
  Mag : Outport
  Phase : Outport  Port=2
  freq : Outport  Port=3
  dfdt : Outport  Port=4
  wires:
  Cartesian to Polar/2 -> Rad->Deg./1, Discrete Derivative/1
  Gain/1 -> Trigonometric Function1/1, Trigonometric Function/1
  t/1 -> Gain/1
  abc/1 -> abc_to_dq0 Transformation/1
  Mux/1 -> abc_to_dq0 Transformation/2
  Discrete Mean value1/1 -> Cartesian to Polar/1  "Real"
  Rad->Deg./1 -> Phase/1
  Discrete Mean value2/1 -> Cartesian to Polar/2  "Real"
  abc_to_dq0 Transformation/1 -> Demux/1
  Demux/3 -> Terminator/1
  Demux/2 -> Discrete Mean value2/1
  Demux/1 -> Discrete Mean value1/1
  Trigonometric Function/1 -> Mux/1
  Trigonometric Function1/1 -> Mux/2
  Cartesian to Polar/1 -> 1 / sqrt of 2/1
  1 / sqrt of 2/1 -> Mag/1
  Discrete Derivative/1 -> Sum/2, dfdt/1
  fo/1 -> Sum/1
  Sum/1 -> freq/1

== system IEEE_39_bus_steady_state/SM_master/PMU_Vpos_60Hz5 ==
  abc : Inport  PortDimensions=3
  1 / sqrt of 2 : Gain  Gain=1/sqrt(2)  OutDataTypeStr=Inherit: Same as input  ParamDataTypeStr=Inherit: Same as input
  Cartesian to Polar : simulink_extras/Transformations/Cartesian to Polar
  Demux : Demux  Outputs=3
      settings: DisplayOption=none
  Discrete Mean value1 : powerlib_extras/Discrete Measurements/Discrete  Mean value  Freq=Freq  Vinit=Real_Init  Ts=Ts
      settings: SourceProductBaseCode=PS
  Discrete Mean value2 : powerlib_extras/Discrete Measurements/Discrete  Mean value  Freq=Freq  Vinit=Imag_Init  Ts=Ts
      settings: SourceProductBaseCode=PS
  Discrete Derivative : simulink/Discrete/Discrete Derivative  gainval=1.0  ICPrevScaledInput=0.0  OutMin=[]  OutMax=[]  OutDataType=fixdt(1, 16)  OutScaling=2^-10  DoSatur=off
  Gain : Gain  Gain=2*pi*Freq  SaturateOnIntegerOverflow=on  OutDataTypeStr=Inherit: Same as input  ParamDataTypeStr=Inherit: Same as input
  Mux : Mux  Inputs=2
  Rad->Deg. : Gain  Gain=180/pi  SaturateOnIntegerOverflow=on  OutDataTypeStr=Inherit: Same as input  ParamDataTypeStr=Inherit: Same as input
  Sum : Sum  Inputs=|++  OutDataTypeStr=Inherit: Same as first input
  Terminator : Terminator
  Trigonometric Function : Trigonometry
  Trigonometric Function1 : Trigonometry  Operator=cos
  abc_to_dq0 Transformation : powerlib_extras/Measurements/abc_to_dq0 Transformation
      settings: SourceProductBaseCode=PS
  fo : Constant  Value=2*pi*Freq
  t : DigitalClock  SampleTime=Ts
  Mag : Outport
  Phase : Outport  Port=2
  freq : Outport  Port=3
  dfdt : Outport  Port=4
  wires:
  Cartesian to Polar/2 -> Rad->Deg./1, Discrete Derivative/1
  Gain/1 -> Trigonometric Function1/1, Trigonometric Function/1
  t/1 -> Gain/1
  abc/1 -> abc_to_dq0 Transformation/1
  Mux/1 -> abc_to_dq0 Transformation/2
  Discrete Mean value1/1 -> Cartesian to Polar/1  "Real"
  Rad->Deg./1 -> Phase/1
  Discrete Mean value2/1 -> Cartesian to Polar/2  "Real"
  abc_to_dq0 Transformation/1 -> Demux/1
  Demux/3 -> Terminator/1
  Demux/2 -> Discrete Mean value2/1
  Demux/1 -> Discrete Mean value1/1
  Trigonometric Function/1 -> Mux/1
  Trigonometric Function1/1 -> Mux/2
  Cartesian to Polar/1 -> 1 / sqrt of 2/1
  1 / sqrt of 2/1 -> Mag/1
  Discrete Derivative/1 -> Sum/2, dfdt/1
  fo/1 -> Sum/1
  Sum/1 -> freq/1

== system IEEE_39_bus_steady_state/SM_master/PMU_Vpos_60Hz6 ==
  abc : Inport  PortDimensions=3
  1 / sqrt of 2 : Gain  Gain=1/sqrt(2)  OutDataTypeStr=Inherit: Same as input  ParamDataTypeStr=Inherit: Same as input
  Cartesian to Polar : simulink_extras/Transformations/Cartesian to Polar
  Demux : Demux  Outputs=3
      settings: DisplayOption=none
  Discrete Mean value1 : powerlib_extras/Discrete Measurements/Discrete  Mean value  Freq=Freq  Vinit=Real_Init  Ts=Ts
      settings: SourceProductBaseCode=PS
  Discrete Mean value2 : powerlib_extras/Discrete Measurements/Discrete  Mean value  Freq=Freq  Vinit=Imag_Init  Ts=Ts
      settings: SourceProductBaseCode=PS
  Discrete Derivative : simulink/Discrete/Discrete Derivative  gainval=1.0  ICPrevScaledInput=0.0  OutMin=[]  OutMax=[]  OutDataType=fixdt(1, 16)  OutScaling=2^-10  DoSatur=off
  Gain : Gain  Gain=2*pi*Freq  SaturateOnIntegerOverflow=on  OutDataTypeStr=Inherit: Same as input  ParamDataTypeStr=Inherit: Same as input
  Mux : Mux  Inputs=2
  Rad->Deg. : Gain  Gain=180/pi  SaturateOnIntegerOverflow=on  OutDataTypeStr=Inherit: Same as input  ParamDataTypeStr=Inherit: Same as input
  Sum : Sum  Inputs=|++  OutDataTypeStr=Inherit: Same as first input
  Terminator : Terminator
  Trigonometric Function : Trigonometry
  Trigonometric Function1 : Trigonometry  Operator=cos
  abc_to_dq0 Transformation : powerlib_extras/Measurements/abc_to_dq0 Transformation
      settings: SourceProductBaseCode=PS
  fo : Constant  Value=2*pi*Freq
  t : DigitalClock  SampleTime=Ts
  Mag : Outport
  Phase : Outport  Port=2
  freq : Outport  Port=3
  dfdt : Outport  Port=4
  wires:
  Cartesian to Polar/2 -> Rad->Deg./1, Discrete Derivative/1
  Gain/1 -> Trigonometric Function1/1, Trigonometric Function/1
  t/1 -> Gain/1
  abc/1 -> abc_to_dq0 Transformation/1
  Mux/1 -> abc_to_dq0 Transformation/2
  Discrete Mean value1/1 -> Cartesian to Polar/1  "Real"
  Rad->Deg./1 -> Phase/1
  Discrete Mean value2/1 -> Cartesian to Polar/2  "Real"
  abc_to_dq0 Transformation/1 -> Demux/1
  Demux/3 -> Terminator/1
  Demux/2 -> Discrete Mean value2/1
  Demux/1 -> Discrete Mean value1/1
  Trigonometric Function/1 -> Mux/1
  Trigonometric Function1/1 -> Mux/2
  Cartesian to Polar/1 -> 1 / sqrt of 2/1
  1 / sqrt of 2/1 -> Mag/1
  Discrete Derivative/1 -> Sum/2, dfdt/1
  fo/1 -> Sum/1
  Sum/1 -> freq/1

== system IEEE_39_bus_steady_state/SM_master/PMU_Vpos_60Hz7 ==
  abc : Inport  PortDimensions=3
  1 / sqrt of 2 : Gain  Gain=1/sqrt(2)  OutDataTypeStr=Inherit: Same as input  ParamDataTypeStr=Inherit: Same as input
  Cartesian to Polar : simulink_extras/Transformations/Cartesian to Polar
  Demux : Demux  Outputs=3
      settings: DisplayOption=none
  Discrete Mean value1 : powerlib_extras/Discrete Measurements/Discrete  Mean value  Freq=Freq  Vinit=Real_Init  Ts=Ts
      settings: SourceProductBaseCode=PS
  Discrete Mean value2 : powerlib_extras/Discrete Measurements/Discrete  Mean value  Freq=Freq  Vinit=Imag_Init  Ts=Ts
      settings: SourceProductBaseCode=PS
  Discrete Derivative : simulink/Discrete/Discrete Derivative  gainval=1.0  ICPrevScaledInput=0.0  OutMin=[]  OutMax=[]  OutDataType=fixdt(1, 16)  OutScaling=2^-10  DoSatur=off
  Gain : Gain  Gain=2*pi*Freq  SaturateOnIntegerOverflow=on  OutDataTypeStr=Inherit: Same as input  ParamDataTypeStr=Inherit: Same as input
  Mux : Mux  Inputs=2
  Rad->Deg. : Gain  Gain=180/pi  SaturateOnIntegerOverflow=on  OutDataTypeStr=Inherit: Same as input  ParamDataTypeStr=Inherit: Same as input
  Sum : Sum  Inputs=|++  OutDataTypeStr=Inherit: Same as first input
  Terminator : Terminator
  Trigonometric Function : Trigonometry
  Trigonometric Function1 : Trigonometry  Operator=cos
  abc_to_dq0 Transformation : powerlib_extras/Measurements/abc_to_dq0 Transformation
      settings: SourceProductBaseCode=PS
  fo : Constant  Value=2*pi*Freq
  t : DigitalClock  SampleTime=Ts
  Mag : Outport
  Phase : Outport  Port=2
  freq : Outport  Port=3
  dfdt : Outport  Port=4
  wires:
  Cartesian to Polar/2 -> Rad->Deg./1, Discrete Derivative/1
  Gain/1 -> Trigonometric Function1/1, Trigonometric Function/1
  t/1 -> Gain/1
  abc/1 -> abc_to_dq0 Transformation/1
  Mux/1 -> abc_to_dq0 Transformation/2
  Discrete Mean value1/1 -> Cartesian to Polar/1  "Real"
  Rad->Deg./1 -> Phase/1
  Discrete Mean value2/1 -> Cartesian to Polar/2  "Real"
  abc_to_dq0 Transformation/1 -> Demux/1
  Demux/3 -> Terminator/1
  Demux/2 -> Discrete Mean value2/1
  Demux/1 -> Discrete Mean value1/1
  Trigonometric Function/1 -> Mux/1
  Trigonometric Function1/1 -> Mux/2
  Cartesian to Polar/1 -> 1 / sqrt of 2/1
  1 / sqrt of 2/1 -> Mag/1
  Discrete Derivative/1 -> Sum/2, dfdt/1
  fo/1 -> Sum/1
  Sum/1 -> freq/1
